simulink library "Mars_Rover_Library"  (R2015a)
settings: Solver=ode45  StartTime=0.0  StopTime=10.0  RelTol=1e-3
libraries: arduinodue_drivers x3, Wheels x2, MarsRover_SimMechanics x2, SingleMotor_Duty_to_inc x2, SingleMotor_V_to_rads x1
settings Model: Creator=tbaroche  LastModifiedBy=tbaroche

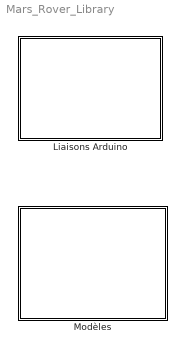
== system Mars_Rover_Library ==
  Liaisons Arduino : Subsystem
  Modèles : Subsystem

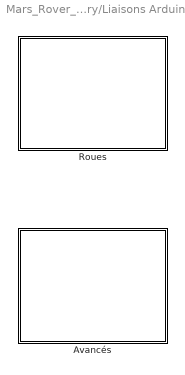
== system Mars_Rover_Library/Liaisons Arduino ==
  Avancés : Subsystem
  Roues : Subsystem

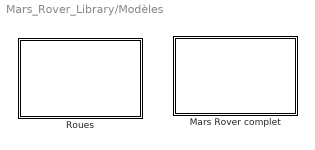
== system Mars_Rover_Library/Modèles ==
  Mars Rover complet : Subsystem
  Roues : Subsystem

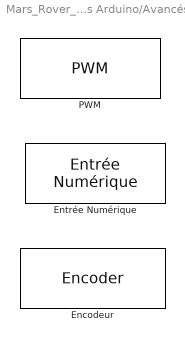
== system Mars_Rover_Library/Liaisons Arduino/Avancés ==
  Encodeur : arduinodue_drivers/Encoder  pinA=18  pinB=19
  Entrée Numérique : arduinodue_drivers/Entrée Numérique  pinNumber=0  isPullUp=on
  PWM : arduinodue_drivers/PWM  pinNumber=2

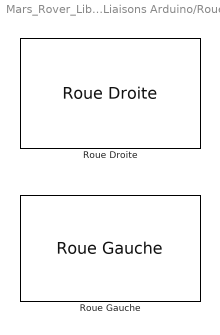
== system Mars_Rover_Library/Liaisons Arduino/Roues ==
  Roue Droite : Wheels/Roue Droite
  Roue Gauche : Wheels/Roue Gauche

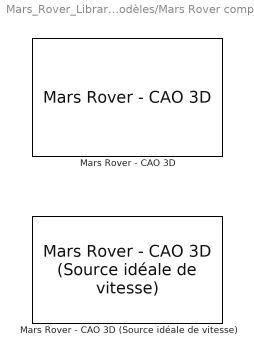
== system Mars_Rover_Library/Modèles/Mars Rover complet ==
  Mars Rover - CAO 3D : MarsRover_SimMechanics/Mars Rover - CAO 3D
  Mars Rover - CAO 3D (Source idéale de vitesse) : MarsRover_SimMechanics/Mars Rover - CAO 3D (Source idéale de vitesse)

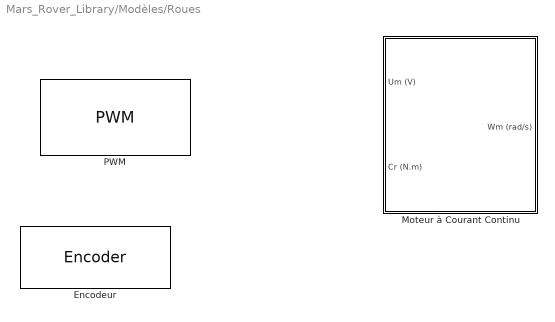
== system Mars_Rover_Library/Modèles/Roues ==
  Encodeur : SingleMotor_Duty_to_inc/Encoder  EncRes=EncRes
  Moteur à Courant Continu : Subsystem  BlockChoice=Modèle Simscape
      link override "SimElectronics Model ": Kphi_lib=Kphi  Rm_lib=Rm  Lm_lib=Lm  bm_lib=bm  Jm_lib=Jm
      settings: AttributesFormatString=%<BlockChoice>  TemplateBlock=SingleMotor_V_to_rads/DC Motor  MemberBlocks=Modèle Simscape,Modèle Simulink
  PWM : SingleMotor_Duty_to_inc/PWM  FreqTriangle=FreqPWM

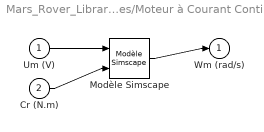
== system Mars_Rover_Library/Modèles/Roues/Moteur à Courant Continu ==
  Um (V) : Inport
  Cr (N.m) : Inport  Port=2
  Modèle Simscape : SingleMotor_V_to_rads/Modèle Simscape  Kphi_lib=Kphi  Rm_lib=Rm  Lm_lib=Lm  bm_lib=bm  Jm_lib=Jm
  Wm (rad/s) : Outport
  wires:
  Um (V)/1 -> Modèle Simscape/1
  Cr (N.m)/1 -> Modèle Simscape/2
  Modèle Simscape/1 -> Wm (rad/s)/1
